simulink model "python_calibration_task"  (Simulink 3.00)
undefined symbols (not defined in the file): acA1920, I32, Long
libraries: mathlib x7, logiclib x2, langlib x1
settings Model: MaskType=REX sequence  MaskIconFrame=on  MaskIconOpaque=on  MaskIconRotate=none  MaskIconUnits=autoscale

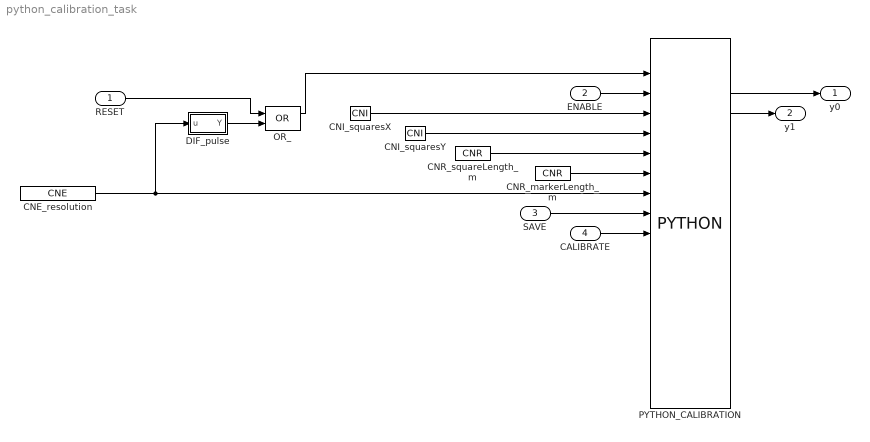
== system python_calibration_task ==
  RESET : Inport  Port=1  OutDataTypeStr=Inherit: auto
  ENABLE : Inport  Port=2  OutDataTypeStr=Inherit: auto
  SAVE : Inport  Port=3  OutDataTypeStr=Inherit: auto
  CALIBRATE : Inport  Port=4  OutDataTypeStr=Inherit: auto
  CNE_resolution : mathlib/CNE  yenum=4: 1920x1080  pupstr=0: 640x480|1: 800x600|2: 1280x720|3: 1280x960|4: 1920x1080|5: 2592x1944
  CNI_squaresX : mathlib/CNI  icn=6  vtype=4: Long (I32)
  CNI_squaresY : mathlib/CNI  icn=6  vtype=4: Long (I32)
  CNR_markerLength_m : mathlib/CNR  ycn=0.055
  CNR_squareLength_m : mathlib/CNR  ycn=0.075
  DIF_pulse : Subsystem  mask(REX sequence){pwidth=2}
  OR_ : logiclib/OR
  PYTHON_CALIBRATION : langlib/PYTHON  srcname=calibration.py  p0=acA1920-40um_23512408.pfs  embedded=on
  y0 : Outport  Port=1  OutDataTypeStr=Inherit: auto
  y1 : Outport  Port=2  OutDataTypeStr=Inherit: auto
  wires:
  CALIBRATE/1 -> PYTHON_CALIBRATION/10
  CNE_resolution/1 -> DIF_pulse/1(u), PYTHON_CALIBRATION/8
  CNI_squaresX/1 -> PYTHON_CALIBRATION/4
  CNI_squaresY/1 -> PYTHON_CALIBRATION/5
  CNR_markerLength_m/1 -> PYTHON_CALIBRATION/7
  CNR_squareLength_m/1 -> PYTHON_CALIBRATION/6
  DIF_pulse/1(Y) -> OR_/2
  ENABLE/1 -> PYTHON_CALIBRATION/3
  OR_/1 -> PYTHON_CALIBRATION/2
  PYTHON_CALIBRATION/3 -> y0/1
  PYTHON_CALIBRATION/4 -> y1/1
  RESET/1 -> OR_/1
  SAVE/1 -> PYTHON_CALIBRATION/9

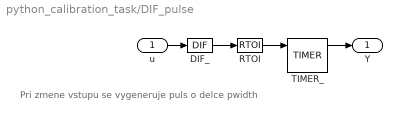
== system python_calibration_task/DIF_pulse ==
  note: Pri zmene vstupu se vygeneruje puls o delce pwidth
  u : Inport  Port=1  OutDataTypeStr=Inherit: auto
  DIF_ : mathlib/DIF  ISSF=on
  RTOI : mathlib/RTOI  vtype=4: Long (I32)  SAT=on
  TIMER_ : logiclib/TIMER  mode=1: Pulse generator  pt=pwidth
  Y : Outport  Port=1  OutDataTypeStr=Inherit: auto
  wires:
  DIF_/1 -> RTOI/1
  RTOI/1 -> TIMER_/1
  TIMER_/1 -> Y/1
  u/1 -> DIF_/1
